simulink model "NetworkReceive1NSP"  (R2016b)
settings: Solver=FixedStepDiscrete  StartTime=0.0  StopTime=inf  FixedStep=sCoreParams.core.stepPeriod  RelTol=1e-3
undefined symbols (not defined in the file): macaddr, sCoreParams
libraries: xpcnetworkbufferlib x4, xpcethernetlib x3, slrtlib x2
settings Model: xpc_rtwmakecfg_data=_xpcetherlib__xpcether8255xlib__xpcetherGbElib__xpciplib__xpcnblib_  Creator=anish  LastModifiedBy=rzelmann
settings SolverCC: EnableConcurrentExecution=on
settings DataIOCC: LimitDataPoints=on  SaveFormat=StructureWithTime  SignalLoggingSaveFormat=ModelDataLogs
settings OptimizationCC: BlockReduction=off  DefaultParameterBehavior=Inlined  OptimizeBlockIOStorage=off  BufferReuse=off  GlobalBufferReuse=off  ExpressionFolding=off  LocalBlockOutputs=off  LifeSpan=inf
settings DebuggingCC: SaveWithParameterizedLinksMsg=none  MultiTaskDSMMsg=warning  MultiTaskCondExecSysMsg=none  StateNameClashWarn=warning  SFUnexpectedBacktrackingDiag=warning  SFNoUnconditionalDefaultTransitionDiag=warning  SFExecutionAtInitializationDiag=none
settings HardwareCC: ProdBitPerPointer=32  ProdBitPerSizeT=32  ProdBitPerPtrDiffT=32  ProdLargestAtomicFloat=None  ProdWordSize=32  ProdLongLongMode=on  ProdHWDeviceType=Generic->32-bit x86 compatible
settings ModelReferenceCC: EnableRefExpFcnMdlSchedulingChecks=off  ModelReferenceNumInstancesAllowed=Single  ModelReferencePassRootInputsByReference=off
settings RTWCC: SystemTargetFile=slrt.tlc  TemplateMakefile=slrt_default_tmf  Description=Simulink Real-Time  RTWCompilerOptimization=on
settings ConfigComp: CovMetricSettings=dw  CovHtmlReporting=on  CovSaveCumulativeToWorkspaceVar=on  CovSaveSingleToWorkspaceVar=on  CovExternalEMLEnable=off

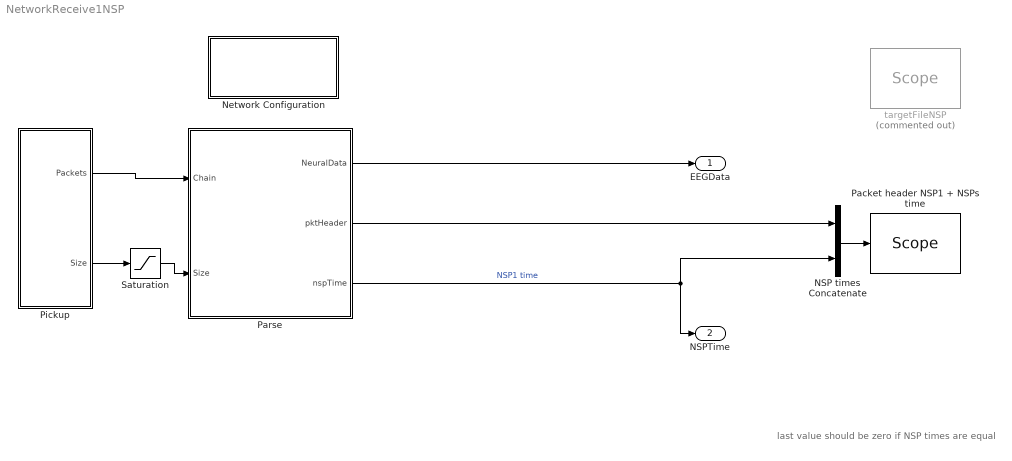
== system NetworkReceive1NSP ==
  note: last value should be zero if NSP times are equal
  NSP times Concatenate : Concatenate
  Network Configuration : Subsystem  mask(xpcnwconfig){IpAddress=192.168.137.7, SubnetMask=255.255.255.0, Gateway=0.0.0.0, EthDrv=Intel Gigabit, PciBus=sCoreParams.network.pciBus(1), PciSlot=sCoreParams.network.pciSlot(1)}
      mask prompts: IpAddress "IP Address:"; SubnetMask "Subnet Mask:"; EthDrv "Ethernet Driver"; PciBus "PCI Bus:"; PciSlot "PCI Slot:"
      mask help: Network Configuration
      mask init:
      | IpAddress = ipaddr(IpAddress);
      | SubnetMask = ipaddr(SubnetMask);
      | Gateway = ipaddr(Gateway);
      mask Help: eval('xpcdoc(''RT_NETWORK_CONFIGURATION'')');
      mask TypeOptions EthDrv: Intel 8255x | Intel Gigabit
      mask Display: disp('Network Configuration');
  Packet header NSP1 + NSPs time : slrtlib/Displays and Logging/Scope   scopeno=1  scopetype=Target  autostart=on  viewmode=Numerical  formatstr='%15.6f'  grid=on  ylimits=[0,0]  nosamples=100  noprepostsamples=0  interleave=1  triggermode=FreeRun  triggersignal=1  trigsignalfromport=off  triggerlevel=0.0  triggerslope=Either  triggerscope=1  triggersample=0  filename=data.dat  mode=Lazy  writesize=512  autorestart=off  dynamicfilemode=off  maxwritefilesize=512*1024^2
  Parse : Subsystem  TreatAsAtomicUnit=on
  Pickup : Subsystem
  Saturation : Saturate  UpperLimit=sCoreParams.network.packetChainSize  LowerLimit=1
  targetFileNSP : slrtlib/Displays and Logging/Scope   Commented=on  scopeno=10  scopetype=File  autostart=on  viewmode=Numerical  formatstr='%15.6f'  grid=on  ylimits=[0,0]  nosamples=1000  noprepostsamples=0  interleave=1  triggermode=FreeRun  triggersignal=1  trigsignalfromport=off  triggerlevel=0.0  triggerslope=Either  triggerscope=1  triggersample=0  filename=NSP1<%%%>.dat  mode=Lazy  writesize=512  autorestart=on  dynamicfilemode=on  maxwritefilesize=512*1024^2
  EEGData : Outport  PortDimensions=[sCoreParams.core.samplesPerStep sCoreParams.core.maxChannelsAllNSPs]  SampleTime=sCoreParams.core.stepPeriod
  NSPTime : Outport  Port=2  PortDimensions=1  SampleTime=sCoreParams.core.stepPeriod
  wires:
  Pickup/1(Packets) -> Parse/1(Chain)
  Pickup/2(Size) -> Saturation/1
  Saturation/1 -> Parse/2(Size)
  Parse/2(pktHeader) -> NSP times Concatenate/1
  Parse/1(NeuralData) -> EEGData/1
  Parse/3(nspTime) -> NSPTime/1, NSP times Concatenate/2  "NSP1 time"
  NSP times Concatenate/1 -> Packet header NSP1 + NSPs time/1

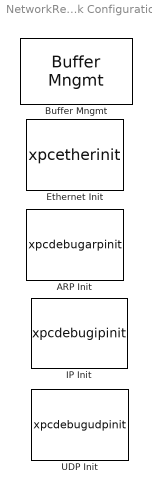
== system NetworkReceive1NSP/Network Configuration ==
  "ARP Init " : S-Function  Priority=0  FunctionName=xpcdebugarpinit  Parameters=Stats, Interface, IpAddress, SubnetMask, Gateway, EthernetId, Flags, BlockId, Retry, Timeout, Expiration, StaticAddressListIp, StaticAddressListMac, DiscoveryList, MulticastList, SampleTime  SFunctionDeploymentMode=off  EnableBusSupport=off  mask(arpinit){Interface=0, IpAddress=IpAddress, SubnetMask=SubnetMask, Gateway=Gateway, EthernetId=1, BlockId=0, SampleTime=-1, Flags=hex2dec('00000697'), Stats=off, Retry=5, Timeout=20, Expiration=20*60, StaticAddressListIp=[], StaticAddressListMac=[], DiscoveryList=[], MulticastList=[]}
      mask prompts: IpAddress "IP Address"; SubnetMask "Subnet Mask"; EthernetId "Ethernet ID"; BlockId "Block ID"; SampleTime "Sample Time"; Stats "Statistics Port"; StaticAddressListIp "[Static IP]"; StaticAddressListMac "[Static MAC]"; DiscoveryList "[Discovery IP]"; MulticastList "[Multicast IP]"
      mask help: ARP Init
      mask init:
      | xpclinklib('xpciplib');
      mask Help: web('arpdebug.htm',  '-helpbrowser');
      mask Display: disp('ARP Init');
  "Buffer Mngmt " : xpcnetworkbufferlib/Buffer Mngmt   Priority=-1  SampleTime=-1  PoolSizes=sCoreParams.network.bufferPoolSizes  ShowTune=off
  "Ethernet Init " : S-Function  Priority=-1  FunctionName=xpcetherinit  Parameters="ID, Driver, Bus, Slot, VendorID, DeviceID, AddressSource, mac, TxSA, RxPromiscuous, RxBad, RxShort, MaxMTU, TxThreshold, TxBuffers, RxBuffers, ShowTune, numMulti, multicast,   NumRxBlks, SampleTime"  SFunctionDeploymentMode=off  EnableBusSupport=off  mask(xpcetherinit){ID=1, Driver=EthDrv, Bus=PciBus, Slot=PciSlot, SampleTime=-1, AddressSource=EEPROM, MAC=macaddr('00:00:00:00:00:00'), TxSA=off, RxPromiscuous=off, Multicast={}, RxBad=off, RxShort=off, MaxMTU=1518, TxThreshold=224, TxBuffers=128, RxBuffers=64, ShowTune=off, NumRxBlks=1}
      mask prompts: ID "Device ID:"; Bus "PCI bus:"; Slot "PCI slot:"; SampleTime "Sample time:"; AddressSource "Address source:"; TxSA "Tx source address from model"; RxPromiscuous "Rx promiscuous"; Multicast "Multicast address list:"; RxBad "Rx bad frames"; RxShort "Rx short frames"; MaxMTU "Max MTU:"; TxThreshold "Tx threshold:"; TxBuffers "Tx buffers:"; RxBuffers "Rx buffers:"; ShowTune "Display tuning information"; NumRxBlks "num rx blocks"
      mask help: Ethernet Initialization
      mask init:
      | VendorID = -1;
      | DeviceID = -1;
      | 
      | [MaskDisplay, VendorID, DeviceID, mac, numMulti, multicast] = mxpcetherinit(2, ID, Driver, Bus, Slot, MAC, Multicast);
      | 
      | set_param(gcb, 'MaskDisplay', MaskDisplay);
      mask Help: eval('xpcdoc(''Ether_Init'')');
      mask TypeOptions ID: 1 | 2 | 3 | 4 | 5 | 6 | 7 | 8
      mask TypeOptions AddressSource: EEPROM | Specify
      mask Callback AddressSource:
      | enables = get_param(gcb, 'MaskVisibilities');
      | if strcmp('Specify', get_param(gcb, 'AddressSource'))
      |     enables{strmatch('MAC',fieldnames(get_param(gcb,'DialogParameters')))} = 'on';
      | else
      |     enables{strmatch('MAC',fieldnames(get_param(gcb,'DialogParameters')))} = 'off';
      | end
      | set_param(gcb, 'MaskVisibilities', enables);
      mask Display: disp('Ethernet\nInitialization\nBus: 4 Slot: 0\nId: 1\nIntel Gigabit');
  "IP Init " : S-Function  Priority=1  FunctionName=xpcdebugipinit  Parameters=Stats, Group, ArpId, IpAddress, SubnetMask, DefaultGateway, DefaultInterface, Flags, ToS, StartingId, TTL, SampleTime  SFunctionDeploymentMode=off  EnableBusSupport=off  mask(ipinit){Group=0, ArpId=[0], IpAddress=[IpAddress], SubnetMask=[SubnetMask], DefaultGateway=Gateway, DefaultInterface=0, SampleTime=-1, Flags=hex2dec('00000005'), ToS=hex2dec('00'), StartingId=10000, TTL=64, Stats=off}
      mask prompts: ArpId "[ARP ID]"; IpAddress "[IP Address]"; SubnetMask "[Subnet Mask]"; DefaultGateway "Default Gateway"; DefaultInterface "Default Interface"; SampleTime "Sample Time"; StartingId "Starting Id"; Stats "Statistics Port"
      mask help: IP Init
      mask init:
      | xpclinklib('xpciplib');
      mask Help: web('ipdebug.htm',  '-helpbrowser');
      mask Display: disp('IP Init');
  "UDP Init " : S-Function  Priority=2  FunctionName=xpcdebugudpinit  Parameters=Stats, Group, StartingPort, Flags, SampleTime  SFunctionDeploymentMode=off  EnableBusSupport=off  mask(udpinit){Group=0, StartingPort=10000, Flags=hex2dec('00000001'), SampleTime=-1, Stats=off}
      mask prompts: StartingPort "Starting Port"; SampleTime "Sample Time"; Stats "Statistics Port"
      mask help: UDP Init
      mask init:
      | xpclinklib('xpciplib');
      mask Help: web('udpdebug.htm',  '-helpbrowser');
      mask Display: disp('UDP Init');

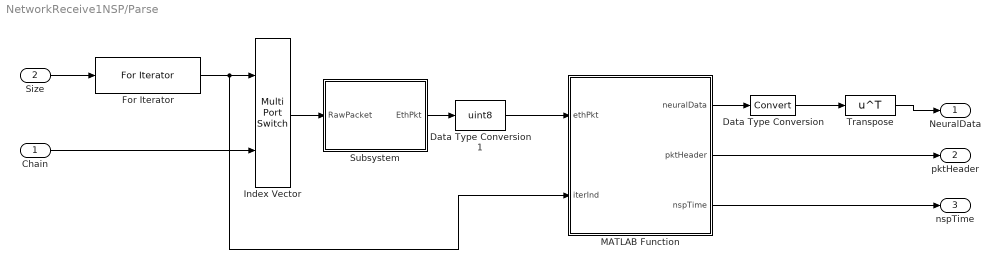
== system NetworkReceive1NSP/Parse ==
  Chain : Inport
  Size : Inport  Port=2
  Data Type Conversion : DataTypeConversion
  Data Type Conversion1 : DataTypeConversion  OutDataTypeStr=uint8
  For Iterator : ForIterator  IterationSource=external  IterationLimit=sCoreParams.network.packetChainSize  IterationVariableDataType=double
  Index Vector : MultiPortSwitch  Inputs=1
  MATLAB Function : MATLAB Function  TreatAsAtomicUnit=on
  Subsystem : Subsystem
  Transpose : Math  Operator=transpose  SaturateOnIntegerOverflow=on
  NeuralData : Outport
  pktHeader : Outport  Port=2
  nspTime : Outport  Port=3
  wires:
  MATLAB Function/1(neuralData) -> Data Type Conversion/1
  Data Type Conversion/1 -> Transpose/1
  Index Vector/1 -> Subsystem/1(RawPacket)
  For Iterator/1 -> MATLAB Function/2(iterInd), Index Vector/1
  Size/1 -> For Iterator/1
  Chain/1 -> Index Vector/2
  Subsystem/1(EthPkt) -> Data Type Conversion1/1
  Transpose/1 -> NeuralData/1
  Data Type Conversion1/1 -> MATLAB Function/1(ethPkt)
  MATLAB Function/2(pktHeader) -> pktHeader/1
  MATLAB Function/3(nspTime) -> nspTime/1

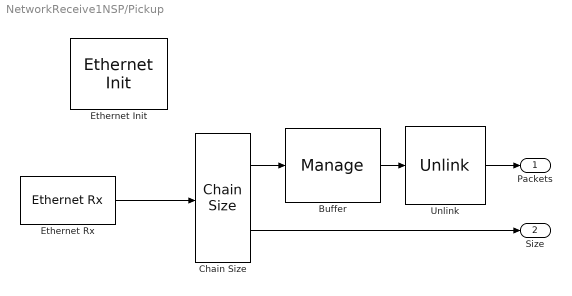
== system NetworkReceive1NSP/Pickup ==
  "Buffer " : xpcnetworkbufferlib/Manage   ChainSize=-sCoreParams.network.packetChainSize  BufferSize=sCoreParams.network.packetChainSize  Threshold=0
  "Chain Size " : xpcnetworkbufferlib/Chain Size 
  "Ethernet Init " : xpcethernetlib/Ethernet Init   Priority=-1  ID=2  Driver=Intel Gigabit  Bus=5  Slot=14  SampleTime=-1  AddressSource=Specify  MAC=macaddr('00:00:00:00:00:00')  TxSA=off  RxPromiscuous=off  Multicast={}  RxBad=off  RxShort=off  MaxMTU=1518  TxThreshold=224  TxBuffers=128  RxBuffers=64  ShowTune=off  NumRxBlks=1
  "Ethernet Rx " : xpcethernetlib/Ethernet Rx   ID=2  SampleTime=sCoreParams.core.stepPeriod  Criteria=Specify types to match  EtherType=[hex2dec('0800')]  BlkID=0
  "Unlink " : xpcnetworkbufferlib/Unlink   VectorLength=sCoreParams.network.packetChainSize
  Packets : Outport
  Size : Outport  Port=2
  wires:
  "Ethernet Rx "/1 -> "Chain Size "/1
  "Chain Size "/1 -> "Buffer "/1
  "Unlink "/1 -> Packets/1
  "Chain Size "/2 -> Size/1
  "Buffer "/1 -> "Unlink "/1

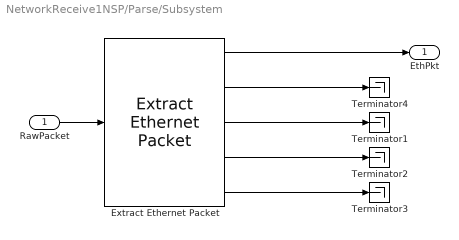
== system NetworkReceive1NSP/Parse/Subsystem ==
  RawPacket : Inport
  "Extract Ethernet Packet " : xpcethernetlib/Extract Ethernet Packet   EthernetDataSize=2048
  Terminator{1..4} (4 alike) : Terminator
  EthPkt : Outport
  wires:
  "Extract Ethernet Packet "/1 -> EthPkt/1
  "Extract Ethernet Packet "/2 -> Terminator4/1
  "Extract Ethernet Packet "/5 -> Terminator3/1
  "Extract Ethernet Packet "/3 -> Terminator1/1
  "Extract Ethernet Packet "/4 -> Terminator2/1
  RawPacket/1 -> "Extract Ethernet Packet "/1

== matlab function NetworkReceive1NSP/Parse/MATLAB Function ==
  data: ethPkt input; neuralData output; iterInd input; pktHeader output; nspTime output
function [neuralData,pktHeader,nspTime]  = PacketParser(ethPkt,iterInd)
%#codegen

%[neuralData,spikeCounts,spikeTimes,pktHeader,nspTime] = PacketParser_EML(ethPkt,iterInd);
%[neuralData,pktHeader,nspTime] = PacketParserBlackRock_EML(ethPkt);
newAcquisition=0; % See if we need to change it when starting new block  
nspTime =0;
%neuralData=zeros(200,2);
[neuralData,pktHeader,nspTime] = PacketParserBlackRock_EML(ethPkt,newAcquisition);
